simulink model "FOUR_bit_even_and_odd_parity_generator"  (R2021b)
settings: Solver=VariableStepAuto  StartTime=0.0  StopTime=1  RelTol=1e-3
settings Model: Creator=Joshua  LastModifiedBy=Joshua

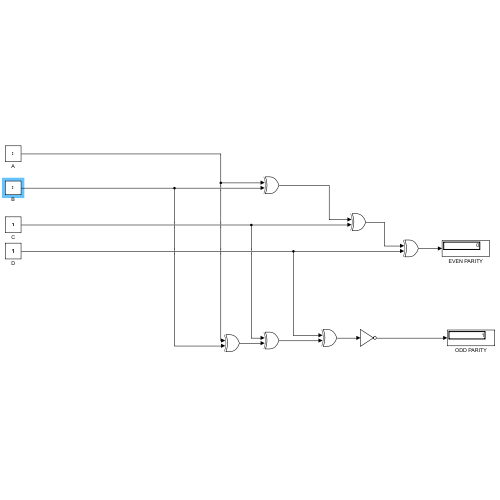
[thumbnail: Simulink's stored preview of the top-level diagram]
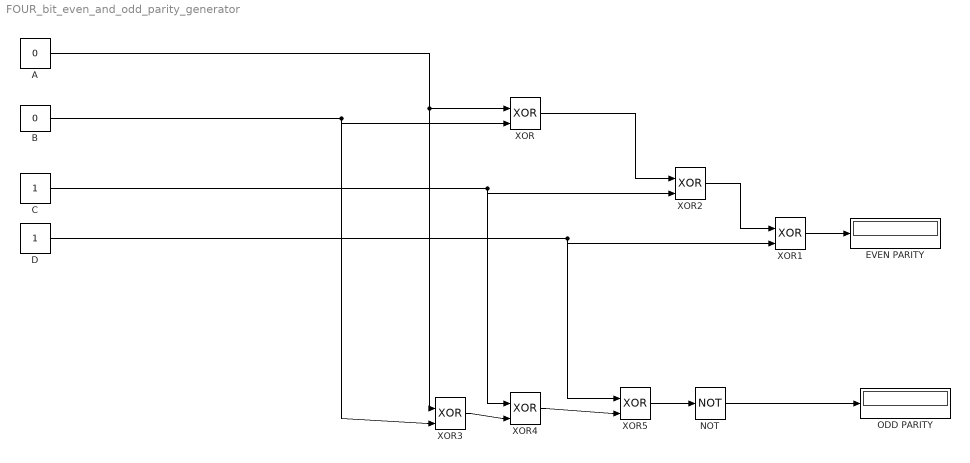
== system FOUR_bit_even_and_odd_parity_generator ==
  A : Constant  Value=0
  B : Constant  Value=0
  C : Constant
  D : Constant
  EVEN PARITY : Display
  NOT : Logic  Operator=NOT  IconShape=distinctive  AllPortsSameDT=off  OutDataTypeStr=boolean
  ODD PARITY : Display
  XOR{,1..5} (6 alike) : Logic  Operator=XOR  IconShape=distinctive  AllPortsSameDT=off  OutDataTypeStr=boolean
  wires:
  B/1 -> XOR3/2, XOR/2
  A/1 -> XOR3/1, XOR/1
  XOR2/1 -> XOR1/1
  D/1 -> XOR1/2, XOR5/1
  XOR1/1 -> EVEN PARITY/1
  XOR/1 -> XOR2/1
  C/1 -> XOR2/2, XOR4/1
  XOR5/1 -> NOT/1
  NOT/1 -> ODD PARITY/1
  XOR4/1 -> XOR5/2
  XOR3/1 -> XOR4/2
